simulink model "PV_MEV"  (R2025a)
settings: Solver=VariableStepAuto  StartTime=0.0  StopTime=1  RelTol=1e-3
InitFcn:
  | init_paras
model workspace (MAT data in the model file):
  atk_params = [0 1 0.85 999 0 50 0 0]
  atk_params_vdc = [0 1 0.85 999 0 50 0 0]
values from neighbouring files (symbols this model uses):
  C_PFC = 2600e-6    (= 0.0026)    [init_paras.m]
  ENABLE_HIL = 0    [init_paras.m]
  estimation_src = 1    [init_paras.m]
  Fnom = 50    [init_paras.m]
  Fr_I = Fnom*2    (= 100)    [init_paras.m]
  Ki_V = 80    [init_paras.m]
  Kp_I = 0.06    [init_paras.m]
  Kp_V = 0.25    [init_paras.m]
  Kr_I = 2.5    [init_paras.m]
  L_PFC = 600e-6    (= 0.0006)    [init_paras.m]
  Limit_V = 100    [init_paras.m]
  mm_10cycle_points = mm_points_per_cycle * 10    (= 800)    [init_paras.m]
  mm_fund_freq = 50    [init_paras.m]
  mm_points_per_cycle = 80    [init_paras.m]
  RL_PFC = 20e-3    (= 0.02)    [init_paras.m]
  Ro = 22.22    [init_paras.m]
  Ts_Control = 1/Fc    (= 5e-05)    [init_paras.m]
  Ts_Power = 50e-9    (= 5e-08)    [init_paras.m]
  use_d_predict = 1    [init_paras.m]
  use_harmonic = 1    [init_paras.m]
  use_p_predict = 0    [init_paras.m]
  Vnom_ac = 240    [init_paras.m]
undefined symbols (not defined in the file or in its folder): D1, Delta, DiscIntNeverNeededParam
libraries: spsSeriesRLCBranchLib x17, spsMeanLib x16, spsCurrentMeasurementLib x9, spsFourierLib x8, spsTHDLib x8, spsVoltageMeasurementLib x8, spsDiodeLib x7, MyLibrary x6, instrumentlib x6, pycoexlib x6, simulink x6, spsPWMGeneratorDCDCLib x4
(part 5 of 6)

== system PV_MEV/EV System1/PFC Control/Speed Regulator2 ==
  note: Anti-windup mechanism: Method of conditionnal integration
      |
      | The integration is suspended if saturation occurs and the
      | control error is of the same sign as the control signal.
      |
      | [1] L.Rundqwist, "Anti-Reset Windup for PID Controllers," Ph.D. Thesis TRFT-1033,
      | Departement of Automatic Control, Lund Institute of Technology, Lund, Sweeden, 1991.
  Vref : Inport  PortDimensions=1
  Vmeas : Inport  Port=2  PortDimensions=1
  Add : Sum  Inputs=+|-
  Compare To Zero : simulink/Logic and Bit Operations/Compare To Zero  relop=>  OutDataTypeStr=uint8  ZeroCross=off
  Compare To Zero1 : simulink/Logic and Bit Operations/Compare To Zero  relop=<  OutDataTypeStr=uint8  ZeroCross=off
  Constant : Constant  Value=0
  Constant1 : Constant  Value=Limit_wreg
  Constant2 : Constant  Value=-Limit_wreg
  Discrete-Time Integrator : DiscreteIntegrator  IntegratorMethod=Integration: Trapezoidal  InitialCondition=Init  SampleTime=Ts  LimitOutput=on  UpperSaturationLimit=Limit_wreg  LowerSaturationLimit=-Limit_wreg  ShowStatePort=on  ICPrevOutput=DiscIntNeverNeededParam  ICPrevScaledInput=DiscIntNeverNeededParam
  Kp4 : Gain  Gain=Kp  SaturateOnIntegerOverflow=on  SampleTime=Ts  OutDataTypeStr=Inherit: Same as input  ParamDataTypeStr=Inherit: Same as input
  Kp5 : Gain  Gain=Ki  SaturateOnIntegerOverflow=on  SampleTime=Ts  OutDataTypeStr=Inherit: Same as input  ParamDataTypeStr=Inherit: Same as input
  Logical Operator : Logic  AllPortsSameDT=off  OutDataTypeStr=boolean
  Logical Operator1 : Logic  AllPortsSameDT=off  OutDataTypeStr=boolean
  Logical Operator2 : Logic  Operator=OR  AllPortsSameDT=off  OutDataTypeStr=boolean
  Relational Operator : RelationalOperator  OutDataTypeStr=boolean  InputSameDT=off
  Relational Operator1 : RelationalOperator  Operator=<=  OutDataTypeStr=boolean  InputSameDT=off
  Saturation2 : Saturate  UpperLimit=Limit_wreg  LowerLimit=-Limit_wreg  SampleTime=Ts
  Sum1 : Sum  InputSameDT=on  SaturateOnIntegerOverflow=on  SampleTime=Ts  OutDataTypeStr=Inherit: Same as first input
  Sum6 : Sum  InputSameDT=on  SaturateOnIntegerOverflow=on  SampleTime=Ts  OutDataTypeStr=Inherit: Same as first input
  Switch : Switch  Criteria=u2 > Threshold  SaturateOnIntegerOverflow=off  InputSameDT=off
  Zero-Order Hold : ZeroOrderHold  SampleTime=Ts
  Out : Outport  SampleTime=Ts  InitialOutput=0  VectorParamsAs1DForOutWhenUnconnected=off
  wires:
  Vmeas/1 -> Add/2
  Vref/1 -> Add/1
  Constant/1 -> Switch/1
  Zero-Order Hold/1 -> Sum1/2, Sum6/1
  Discrete-Time Integrator/State -> Sum1/1
  Sum1/1 -> Relational Operator1/1, Relational Operator/1
  Logical Operator2/1 -> Switch/2
  Relational Operator/1 -> Logical Operator/1  "UpperLimit_is_Reached"
  Relational Operator1/1 -> Logical Operator1/1  "LowerLimit_Is_Reached"
  Constant1/1 -> Relational Operator/2
  Constant2/1 -> Relational Operator1/2
  Compare To Zero/1 -> Logical Operator/2  "Error_is_positive"
  Logical Operator/1 -> Logical Operator2/1
  Logical Operator1/1 -> Logical Operator2/2
  Compare To Zero1/1 -> Logical Operator1/2  "Error_is_negative"
  Add/1 -> Kp4/1, Kp5/1, Compare To Zero1/1, Compare To Zero/1
  Sum6/1 -> Saturation2/1
  Kp4/1 -> Zero-Order Hold/1
  Discrete-Time Integrator/1 -> Sum6/2
  Saturation2/1 -> Out/1
  Switch/1 -> Discrete-Time Integrator/1
  Kp5/1 -> Switch/3

== system PV_MEV/EV System1/PFC Control/fft estimation 1 cycle2 ==
  u : Inport
  Buffer 1cycle : Buffer  N=mm_points_per_cycle  V=mm_sampling_overlap  OutputFrames=off
  Constant4 : Constant  Value=mm_fund_freq
  Constant5 : Constant  Value=mm_points_per_cycle * mm_fund_freq
  FFT_estimation_1 : MATLAB Function  TreatAsAtomicUnit=on
  Sampling : ZeroOrderHold  SampleTime=1/(mm_fund_freq*mm_points_per_cycle)
  amp : Outport
  phase : Outport  Port=2
  wires:
  FFT_estimation_1/2(phase) -> phase/1
  FFT_estimation_1/1(amp) -> amp/1
  u/1 -> Sampling/1
  Constant4/1 -> FFT_estimation_1/3(f0)
  Constant5/1 -> FFT_estimation_1/2(fs)
  Buffer 1cycle/1 -> FFT_estimation_1/1(u)
  Sampling/1 -> Buffer 1cycle/1

== system PV_MEV/EV System1/PFC Control/fft estimation 10 cycle2 ==
  u : Inport
  Buffer 10cycle : Buffer  N=mm_10cycle_points  V=mm_10cycle_overlap  OutputFrames=off
  Constant4 : Constant  Value=mm_fund_freq
  Constant5 : Constant  Value=mm_points_per_cycle * mm_fund_freq
  FFT_estimation : MATLAB Function  TreatAsAtomicUnit=on
  Sampling : ZeroOrderHold  SampleTime=1/(mm_fund_freq*mm_points_per_cycle)
  amp : Outport
  phase : Outport  Port=2
  wires:
  Sampling/1 -> Buffer 10cycle/1
  Buffer 10cycle/1 -> FFT_estimation/1(u)
  Constant5/1 -> FFT_estimation/2(fs)
  Constant4/1 -> FFT_estimation/3(f0)
  u/1 -> Sampling/1
  FFT_estimation/1(amp) -> amp/1
  FFT_estimation/2(phase) -> phase/1

== system PV_MEV/EV System2/PFC Control/Half Cycle Model Prediction ==
  u : Inport
  Constant1 : Constant  Value=0.01
  Data Type Conversion : DataTypeConversion  SaturateOnIntegerOverflow=off  RndMeth=Floor
  Data Type Conversion1 : DataTypeConversion  SaturateOnIntegerOverflow=off  RndMeth=Floor
  Data Type Conversion2 : DataTypeConversion  SaturateOnIntegerOverflow=off  RndMeth=Floor
  Demux : Demux  Outputs=7
  MATLAB Function : MATLAB Function  TreatAsAtomicUnit=on
  MATLAB Function3 : MATLAB Function  TreatAsAtomicUnit=on
  Mux1 : Mux  Inputs=3
  Mux6 : Mux
  ONNX Model Predict : pycoexlib/ONNX Model Predict  ModelFile=/home/changhong/prj/finn_cli_fork/scripts/HIL/HarmonicAI_Simulation/Model_Training2/harmonic_brevitas_run_half_opt/brevitas_harmonic_mlp.onnx  ExecutionProviders=CPUExecutionProvider  InputTable={ 'input', 'float32', '', '2' }  OutputTable={ 'output', '', '' }  SampleTime=1/2000  InputDatatypes=float32  InputNumDims=2  InputPermutations=[]  OutputPermutations=[]  PythonCoexecutionBlockType=ONNXModelBlock  VariableOutputMaxSizes=[]
  Sampling1 : ZeroOrderHold  SampleTime=1/2000
  Transpose : Math  Operator=transpose
  u_buff : Buffer  N=40  V=39  OutputFrames=off
  amplitude : Outport
  phase : Outport  Port=2
  wires:
  Transpose/1 -> MATLAB Function/1(x)
  u_buff/1 -> Transpose/1
  u/1 -> Sampling1/1
  Mux1/1 -> phase/1
  Mux6/1 -> amplitude/1
  Data Type Conversion2/1 -> Demux/1
  MATLAB Function3/1(y_post) -> Data Type Conversion2/1
  Demux/1 -> Mux6/1
  Demux/2 -> Mux6/2
  Demux/3 -> Mux6/3
  Demux/4 -> Mux6/4
  Demux/5 -> Mux1/1
  Demux/6 -> Mux1/2
  Demux/7 -> Mux1/3
  MATLAB Function/2(A) -> MATLAB Function3/2(A_latest)
  Constant1/1 -> MATLAB Function3/3(alpha)
  Data Type Conversion1/1 -> MATLAB Function3/1(y_rel)
  ONNX Model Predict/1 -> Data Type Conversion1/1
  Data Type Conversion/1 -> ONNX Model Predict/1
  MATLAB Function/1(x_norm) -> Data Type Conversion/1
  Sampling1/1 -> u_buff/1

== system PV_MEV/EV System2/PFC Control/One  Cycle Model Prediction ==
  u : Inport
  Constant1 : Constant  Value=0.05
  Data Type Conversion : DataTypeConversion  SaturateOnIntegerOverflow=off  RndMeth=Floor
  Data Type Conversion1 : DataTypeConversion  SaturateOnIntegerOverflow=off  RndMeth=Floor
  Data Type Conversion2 : DataTypeConversion  SaturateOnIntegerOverflow=off  RndMeth=Floor
  Demux : Demux  Outputs=7
  MATLAB Function : MATLAB Function  TreatAsAtomicUnit=on
  MATLAB Function3 : MATLAB Function  TreatAsAtomicUnit=on
  Mux1 : Mux  Inputs=3
  Mux6 : Mux
  ONNX Model Predict : pycoexlib/ONNX Model Predict  ModelFile=/home/changhong/prj/finn_cli_fork/scripts/HIL/HarmonicAI_Simulation/Model_Training2/harmonic_brevitas_run_1cycle/brevitas_harmonic_mlp.onnx  ExecutionProviders=AzureExecutionProvider, CPUExecutionProvider  InputTable={ 'input', 'float32', '', '2' }  OutputTable={ 'output', '', '' }  SampleTime=1/4000  InputDatatypes=float32  InputNumDims=2  InputPermutations=[]  OutputPermutations=[]  PythonCoexecutionBlockType=ONNXModelBlock  VariableOutputMaxSizes=[]
  Sampling1 : ZeroOrderHold  SampleTime=1/(mm_fund_freq*mm_points_per_cycle)
  Transpose : Math  Operator=transpose
  u_buff : Buffer  N=mm_points_per_cycle  V=mm_sampling_overlap  OutputFrames=off
  amplitude : Outport
  phase : Outport  Port=2
  wires:
  Sampling1/1 -> u_buff/1
  MATLAB Function/1(x_norm) -> Data Type Conversion/1
  Data Type Conversion/1 -> ONNX Model Predict/1
  ONNX Model Predict/1 -> Data Type Conversion1/1
  Data Type Conversion1/1 -> MATLAB Function3/1(y_rel)
  Constant1/1 -> MATLAB Function3/3(alpha)
  MATLAB Function/2(A) -> MATLAB Function3/2(A_latest)
  Demux/7 -> Mux1/3
  Demux/6 -> Mux1/2
  Demux/5 -> Mux1/1
  Demux/4 -> Mux6/4
  Demux/3 -> Mux6/3
  Demux/2 -> Mux6/2
  Demux/1 -> Mux6/1
  MATLAB Function3/1(y_post) -> Data Type Conversion2/1
  Data Type Conversion2/1 -> Demux/1
  Mux6/1 -> amplitude/1
  Mux1/1 -> phase/1
  u/1 -> Sampling1/1
  u_buff/1 -> Transpose/1
  Transpose/1 -> MATLAB Function/1(x)

== system PV_MEV/EV System2/PFC Control/PR2 ==
  Iref : Inport
  Iac : Inport  Port=2
  Gain : Gain  Gain=Kp
  Gain1 : Gain  Gain=Kr
  Second-Order Filter1 : spsSecondOrderFilterLib/Second-Order Filter  FilterType=Bandpass  Fo=Fr  Zeta=Zeta_I  Ts=Ts_Control  Initialize=off  Vac_Init="[0,  0,  60]"  Vdc_Init=0  PlotResponse=off  FreqRange=[0, 1000, 0.2]
  Sum1 : Sum  Inputs=|+-
  Sum2 : Sum  Inputs=|++
  D : Outport
  wires:
  Gain1/1 -> Second-Order Filter1/1
  Sum2/1 -> D/1
  Gain/1 -> Sum2/1
  Iac/1 -> Sum1/2
  Iref/1 -> Sum1/1
  Sum1/1 -> Gain1/1, Gain/1
  Second-Order Filter1/1 -> Sum2/2

== system PV_MEV/EV System2/PFC Control/Speed Regulator2 ==
  note: Anti-windup mechanism: Method of conditionnal integration
      |
      | The integration is suspended if saturation occurs and the
      | control error is of the same sign as the control signal.
      |
      | [1] L.Rundqwist, "Anti-Reset Windup for PID Controllers," Ph.D. Thesis TRFT-1033,
      | Departement of Automatic Control, Lund Institute of Technology, Lund, Sweeden, 1991.
  Vref : Inport  PortDimensions=1
  Vmeas : Inport  Port=2  PortDimensions=1
  Add : Sum  Inputs=+|-
  Compare To Zero : simulink/Logic and Bit Operations/Compare To Zero  relop=>  OutDataTypeStr=uint8  ZeroCross=off
  Compare To Zero1 : simulink/Logic and Bit Operations/Compare To Zero  relop=<  OutDataTypeStr=uint8  ZeroCross=off
  Constant : Constant  Value=0
  Constant1 : Constant  Value=Limit_wreg
  Constant2 : Constant  Value=-Limit_wreg
  Discrete-Time Integrator : DiscreteIntegrator  IntegratorMethod=Integration: Trapezoidal  InitialCondition=Init  SampleTime=Ts  LimitOutput=on  UpperSaturationLimit=Limit_wreg  LowerSaturationLimit=-Limit_wreg  ShowStatePort=on  ICPrevOutput=DiscIntNeverNeededParam  ICPrevScaledInput=DiscIntNeverNeededParam
  Kp4 : Gain  Gain=Kp  SaturateOnIntegerOverflow=on  SampleTime=Ts  OutDataTypeStr=Inherit: Same as input  ParamDataTypeStr=Inherit: Same as input
  Kp5 : Gain  Gain=Ki  SaturateOnIntegerOverflow=on  SampleTime=Ts  OutDataTypeStr=Inherit: Same as input  ParamDataTypeStr=Inherit: Same as input
  Logical Operator : Logic  AllPortsSameDT=off  OutDataTypeStr=boolean
  Logical Operator1 : Logic  AllPortsSameDT=off  OutDataTypeStr=boolean
  Logical Operator2 : Logic  Operator=OR  AllPortsSameDT=off  OutDataTypeStr=boolean
  Relational Operator : RelationalOperator  OutDataTypeStr=boolean  InputSameDT=off
  Relational Operator1 : RelationalOperator  Operator=<=  OutDataTypeStr=boolean  InputSameDT=off
  Saturation2 : Saturate  UpperLimit=Limit_wreg  LowerLimit=-Limit_wreg  SampleTime=Ts
  Sum1 : Sum  InputSameDT=on  SaturateOnIntegerOverflow=on  SampleTime=Ts  OutDataTypeStr=Inherit: Same as first input
  Sum6 : Sum  InputSameDT=on  SaturateOnIntegerOverflow=on  SampleTime=Ts  OutDataTypeStr=Inherit: Same as first input
  Switch : Switch  Criteria=u2 > Threshold  SaturateOnIntegerOverflow=off  InputSameDT=off
  Zero-Order Hold : ZeroOrderHold  SampleTime=Ts
  Out : Outport  SampleTime=Ts  InitialOutput=0  VectorParamsAs1DForOutWhenUnconnected=off
  wires:
  Kp5/1 -> Switch/3
  Switch/1 -> Discrete-Time Integrator/1
  Saturation2/1 -> Out/1
  Discrete-Time Integrator/1 -> Sum6/2
  Kp4/1 -> Zero-Order Hold/1
  Sum6/1 -> Saturation2/1
  Add/1 -> Compare To Zero/1, Compare To Zero1/1, Kp5/1, Kp4/1
  Compare To Zero1/1 -> Logical Operator1/2  "Error_is_negative"
  Logical Operator1/1 -> Logical Operator2/2
  Logical Operator/1 -> Logical Operator2/1
  Compare To Zero/1 -> Logical Operator/2  "Error_is_positive"
  Constant2/1 -> Relational Operator1/2
  Constant1/1 -> Relational Operator/2
  Relational Operator1/1 -> Logical Operator1/1  "LowerLimit_Is_Reached"
  Relational Operator/1 -> Logical Operator/1  "UpperLimit_is_Reached"
  Logical Operator2/1 -> Switch/2
  Sum1/1 -> Relational Operator/1, Relational Operator1/1
  Discrete-Time Integrator/State -> Sum1/1
  Zero-Order Hold/1 -> Sum6/1, Sum1/2
  Constant/1 -> Switch/1
  Vref/1 -> Add/1
  Vmeas/1 -> Add/2

== system PV_MEV/EV System2/PFC Control/fft estimation 1 cycle2 ==
  u : Inport
  Buffer 1cycle : Buffer  N=mm_points_per_cycle  V=mm_sampling_overlap  OutputFrames=off
  Constant4 : Constant  Value=mm_fund_freq
  Constant5 : Constant  Value=mm_points_per_cycle * mm_fund_freq
  FFT_estimation_1 : MATLAB Function  TreatAsAtomicUnit=on
  Sampling : ZeroOrderHold  SampleTime=1/(mm_fund_freq*mm_points_per_cycle)
  amp : Outport
  phase : Outport  Port=2
  wires:
  Sampling/1 -> Buffer 1cycle/1
  Buffer 1cycle/1 -> FFT_estimation_1/1(u)
  Constant5/1 -> FFT_estimation_1/2(fs)
  Constant4/1 -> FFT_estimation_1/3(f0)
  u/1 -> Sampling/1
  FFT_estimation_1/1(amp) -> amp/1
  FFT_estimation_1/2(phase) -> phase/1

== system PV_MEV/EV System2/PFC Control/fft estimation 10 cycle2 ==
  u : Inport
  Buffer 10cycle : Buffer  N=mm_10cycle_points  V=mm_10cycle_overlap  OutputFrames=off
  Constant4 : Constant  Value=mm_fund_freq
  Constant5 : Constant  Value=mm_points_per_cycle * mm_fund_freq
  FFT_estimation : MATLAB Function  TreatAsAtomicUnit=on
  Sampling : ZeroOrderHold  SampleTime=1/(mm_fund_freq*mm_points_per_cycle)
  amp : Outport
  phase : Outport  Port=2
  wires:
  FFT_estimation/2(phase) -> phase/1
  FFT_estimation/1(amp) -> amp/1
  u/1 -> Sampling/1
  Constant4/1 -> FFT_estimation/3(f0)
  Constant5/1 -> FFT_estimation/2(fs)
  Buffer 10cycle/1 -> FFT_estimation/1(u)
  Sampling/1 -> Buffer 10cycle/1

== system PV_MEV/PV System/DC AC Inverter/VSC Control ==
  note: VSC Main Controller
  Vabc_prim : Inport  PortDimensions=3
  Iabc_prim : Inport  Port=2  PortDimensions=3
  Vdc_mes : Inport  Port=3  PortDimensions=1
  Current Regulator : Subsystem
  Iq_ref : Constant  Value=0
  Mux : Mux  Inputs=2
  PLL & Measurements : Subsystem
  PWM Generator (3-Level) : spsPWMGenerator3LevelLib/PWM Generator (3-Level)  ModulatorType=Three-phase bridge (12 pulses)  ModulatorMode=Unsynchronized  nF=27  Fc=33*60  ModulatingSignals=off  m=0.8  Freq=60  Phase=0  Ts=Ts_Power
  Uabc_ref Generation max (m) = 1 : Subsystem
  Unit Delay : UnitDelay  SampleTime=Ts_Control  HasFrameUpgradeWarning=on
  VDC Regulator : Subsystem
  Vdc_ref1 : Constant  Value=Vdc_ref
  Pulses : Outport  VectorParamsAs1DForOutWhenUnconnected=off
  wires:
  VDC Regulator/1(Id_ref) -> Mux/1
  PLL & Measurements/1(wt) -> Uabc_ref Generation max (m) = 1/1(wt)
  Current Regulator/1(VdVq_conv) -> Uabc_ref Generation max (m) = 1/2(VdVq_conv)
  Iq_ref/1 -> Mux/2
  Mux/1 -> Current Regulator/3(IdIq_ref)
  PLL & Measurements/3(IdIq_prim) -> Current Regulator/2(IdIq_mes)
  PLL & Measurements/2(VdVq_prim) -> Current Regulator/1(VdVq_mes)
  Vdc_mes/1 -> VDC Regulator/1(Vdc_mes)
  Vabc_prim/1 -> PLL & Measurements/1(Vabc_prim)
  Iabc_prim/1 -> PLL & Measurements/2(Iabc_prim)
  Unit Delay/1 -> PWM Generator (3-Level)/1
  PWM Generator (3-Level)/1 -> Pulses/1
  Uabc_ref Generation max (m) = 1/1(Uabc_ref) -> Unit Delay/1
  Vdc_ref1/1 -> VDC Regulator/2(Vdc_ref)

== system PV_MEV/PV System/DC DC Boost Converter/MPPT Controller using  'Incremental Conductance + Integral Regulator'  technique  ==
  V_PV : Inport
  I_PV : Inport  Port=2
  Add : Sum  Inputs=+-
  Deblock MPPT : Step  Time=0.4  SampleTime=0
  Duty Cycle : Constant  Value=Dinit
  MPPT : Subsystem
  PWM Generator (DC-DC) : spsPWMGeneratorDCDCLib/PWM Generator (DC-DC)  Fsw=fc  Ts=Ts_Power
  Saturation : Saturate  UpperLimit=1  LowerLimit=0
  Pulses : Outport  VectorParamsAs1DForOutWhenUnconnected=off
  tag scope: D=global
  wires:
  V_PV/1 -> MPPT/1(V_PV)
  I_PV/1 -> MPPT/2(I_PV)
  PWM Generator (DC-DC)/1 -> Pulses/1
  Deblock MPPT/1 -> MPPT/3(on/off)
  Saturation/1 -> PWM Generator (DC-DC)/1, [D]
  Add/1 -> Saturation/1  "D"
  MPPT/1(Delta_D) -> Add/2
  Duty Cycle/1 -> Add/1

== system PV_MEV/PV System/DC AC Inverter/VSC Control/Current Regulator ==
  note: harmonic filter neglected
  note: Vd_mes + Id*R - Iq*L + deriv(Id)*L= Vd_conv
  note: Vq_mes + Id*L + Iq*R + deriv(Iq)*L= Vq_conv
  note: Current Regulator
      | (with feedforward)
  note: Sign Convention: Current going out of the converter = positive current
  note: Iq positive --> The converter absorbs reactive power ("Inductive mode") = Reactive Power Q negative
  note: Id positive --> The converter generates active power ("Inverter mode") = Active Power P positive
  note: Ltot = Lxfo + Lchoke
      | Rtot = Rxfo + Rchoke
  note: (Vd_prim - Vd_conv) ~= + Iq * Ltot
  note: (Vq_prim - Vq_conv) ~ = - Id * Ltot
  note: For Ltot >> Rtot :
  VdVq_mes : Inport  PortDimensions=2
  IdIq_mes : Inport  Port=2  PortDimensions=2
  IdIq_ref : Inport  Port=3  PortDimensions=2
  Add1 : Sum  Inputs=++-
  Add2 : Sum
  Add3 : Sum  Inputs=+++
  Demux : Demux  Outputs=2
  Demux1 : Demux  Outputs=2
  Ltot_pu1 : Gain  Gain=Ltot_pu  SaturateOnIntegerOverflow=on  OutDataTypeStr=Inherit: Same as input  ParamDataTypeStr=Inherit: Same as input
  Ltot_pu2 : Gain  Gain=Ltot_pu  SaturateOnIntegerOverflow=on  OutDataTypeStr=Inherit: Same as input  ParamDataTypeStr=Inherit: Same as input
  Mux : Mux  Inputs=2
  PI : slpidlib/PID Controller  Controller=PI  Form=Parallel  TimeDomain=Discrete-time  UseExternalTs=off  SampleTime=Ts  IntegratorMethod=Forward Euler  FilterMethod=Forward Euler  ControllerParametersSource=internal  P=Kp_Ireg  I=Ki_Ireg  UseKiTs=off  D=0  UseExternalDerivativeSource=off  N=100  UseFilter=on  TunerSelectOption=Transfer Function Based (PID Tuner App)  InitialConditionSource=internal  InitialConditionForIntegrator=0  InitialConditionForFilter=0  DifferentiatorICPrevScaledInput=0  ExternalReset=none  TrackingMode=off  Kt=1  LimitOutput=on  SatLimitsSource=internal  UpperSaturationLimit=2  LowerSaturationLimit=-2  LinearizeAsGain=off  AntiWindupMode=none  Kb=1  LimitIntegrator=off  UpperIntegratorSaturationLimit=inf  LowerIntegratorSaturationLimit=-inf  POutMin=[]  POutMax=[]  IOutMin=[]  IOutMax=[]  DOutMin=[]  DOutMax=[]  NOutMin=[]  NOutMax=[]  SumOutMin=[]  SumOutMax=[]  SaturationOutMin=[]  SaturationOutMax=[]  PParamMin=[]  PParamMax=[]  IParamMin=[]  IParamMax=[]  DParamMin=[]  DParamMax=[]  NParamMin=[]  NParamMax=[]  KbParamMin=[]  KbParamMax=[]  KtParamMin=[]  KtParamMax=[]  KbOutMin=[]  KbOutMax=[]  KtOutMin=[]  KtOutMax=[]  IntegratorOutMin=[]  IntegratorOutMax=[]  FilterOutMin=[]  FilterOutMax=[]  SumI1OutMin=[]  SumI1OutMax=[]  SumI2OutMin=[]  SumI2OutMax=[]  SumI3OutMin=[]  SumI3OutMax=[]  SumI4OutMin=[]  SumI4OutMax=[]  SumDOutMin=[]  SumDOutMax=[]  DifferentiatorOutMin=[]  DifferentiatorOutMax=[]  FilterDiffOutCoefMin=[]  FilterDiffOutCoefMax=[]  ReciprocalOutMin=[]  ReciprocalOutMax=[]  SumDenOutMin=[]  SumDenOutMax=[]  SumNumOutMin=[]  SumNumOutMax=[]  DivideOutMin=[]  DivideOutMax=[]  UdiffTsProdOutMin=[]  UdiffTsProdOutMax=[]  NTsProdOutMin=[]  NTsProdOutMax=[]  UintegralTsProdOutMin=[]  UintegralTsProdOutMax=[]  UngainTsProdOutMin=[]  UngainTsProdOutMax=[]  ClampingZeroOutDataTypeStr=Inherit: Inherit via back propagation  ClampingZeroOutMin=[]  ClampingZeroOutMax=[]  FilterDenConstantOutDataTypeStr=Inherit: Inherit via back propagation  FilterDenConstantOutMin=[]  FilterDenConstantOutMax=[]  PCopyOutDataTypeStr=Inherit: Inherit via back propagation  PCopyOutMin=[]  PCopyOutMax=[]  NCopyOutDataTypeStr=Inherit: Inherit via back propagation  NCopyOutMin=[]  NCopyOutMax=[]  IntegratorContinuousStateAttributes=''  IntegratorStateMustResolveToSignalObject=off  IntegratorRTWStateStorageClass=Auto  FilterContinuousStateAttributes=''  FilterStateMustResolveToSignalObject=off  FilterRTWStateStorageClass=Auto  ParallelPVariant=InternalParameters  IdealPVariant=Disabled  IVariant=InternalParameters  DVariant=Disabled  IntegratorVariant=Discrete  SatVariant=Enabled  AWVariant=Passthrough  PCopyVariant=Disabled  TRVariant=Disabled  FdbkBlocksVariant=Forward  IdealPFdbkVariant=Disabled  SatFdbkVariant=Disabled  DerivativeFilterVariant=Disabled  NVariant=Disabled  NCopyVariant=Disabled_SignalSpec  FilterICVariant=Disabled  IntegratorICVariant=InternalICs  ExternalResetVariant=Disabled  TRSumVariant=Passthrough  SumFdbkVariant=Disabled  SumVariant=Sum_PI  TsampFilterVariant=InternalTs  TsampNgainVariant=Passthrough  TsampIntegralVariant=Disabled_SignalSpec  ExternalSaturationOutDataTypeStr=Inherit: Same as second input  DerivativeSourceVariant=Disabled  PreIntVariant=InternalPreInt
  PI_Ireg1 : Scope
      settings: DataLoggingSaveFormat=Array
  Rtot_pu1 : Gain  Gain=Rtot_pu  SaturateOnIntegerOverflow=on  OutDataTypeStr=Inherit: Same as input  ParamDataTypeStr=Inherit: Same as input
  Rtot_pu5 : Gain  Gain=Rtot_pu  SaturateOnIntegerOverflow=on  OutDataTypeStr=Inherit: Same as input  ParamDataTypeStr=Inherit: Same as input
  Saturation : Saturate  UpperLimit=2  LowerLimit=-2
  Sum : Sum  Inputs=|-+
  VdVq_conv : Outport  VectorParamsAs1DForOutWhenUnconnected=off
  wires:
  Mux/1 -> PI_Ireg1/1, Add2/2
  PI/1 -> Add2/1  "PI"
  Sum/1 -> PI/1
  IdIq_ref/1 -> Sum/2, Demux1/1
  IdIq_mes/1 -> Sum/1
  Add2/1 -> Saturation/1
  Saturation/1 -> VdVq_conv/1
  VdVq_mes/1 -> Demux/1
  Demux/1 -> Add1/1
  Rtot_pu1/1 -> Add1/2
  Demux1/1 -> Rtot_pu1/1, Ltot_pu2/1
  Ltot_pu1/1 -> Add1/3
  Demux1/2 -> Ltot_pu1/1, Rtot_pu5/1
  Rtot_pu5/1 -> Add3/2
  Ltot_pu2/1 -> Add3/3
  Add1/1 -> Mux/1  "Feedforward"
  Demux/2 -> Add3/1
  Add3/1 -> Mux/2

== system PV_MEV/PV System/DC AC Inverter/VSC Control/PLL & Measurements ==
  Vabc_prim : Inport
  Iabc_prim : Inport  Port=2
  PLL (3ph) : spsPLL3phLib/PLL (3ph)  Fmin=45  Par_Init="[-0.57  Fnom]"  ParK=[180, 3200, 1]  TcD=1e-4  MaxRateChangeFreq=12  FilterCutOffFreq=25  Ts=Ts  AGC=on
  Selector1 : Selector  InputPortWidth=3  IndexOptions=Index vector (dialog)  Indices=[1 2]  OutputSizes=1
  Selector2 : Selector  InputPortWidth=3  IndexOptions=Index vector (dialog)  Indices=[1 2]  OutputSizes=1
  Terminator : Terminator
  V->pu : Gain  Gain=1/(Vnom_prim*sqrt(2)/sqrt(3))  SaturateOnIntegerOverflow=on  OutDataTypeStr=Inherit: Same as input  ParamDataTypeStr=Inherit: Same as input
  V->pu1 : Gain  Gain=Vnom_prim*sqrt(3)/Pnom/sqrt(2)  SaturateOnIntegerOverflow=on  OutDataTypeStr=Inherit: Same as input  ParamDataTypeStr=Inherit: Same as input
  abc to dq0 : spsabctodq0Lib/abc to dq0  Alignment=90 degrees behind phase A axis
  abc to dq1 : spsabctodq0Lib/abc to dq0  Alignment=90 degrees behind phase A axis
  wt : Outport  VectorParamsAs1DForOutWhenUnconnected=off
  VdVq_prim : Outport  Port=2  VectorParamsAs1DForOutWhenUnconnected=off
  IdIq_prim : Outport  Port=3  VectorParamsAs1DForOutWhenUnconnected=off
  tag scope: IdIq_prim=global
  wires:
  V->pu1/1 -> abc to dq1/1
  V->pu/1 -> PLL (3ph)/1, abc to dq0/1
  abc to dq1/1 -> Selector1/1
  Vabc_prim/1 -> V->pu/1
  Iabc_prim/1 -> V->pu1/1
  abc to dq0/1 -> Selector2/1
  Selector2/1 -> VdVq_prim/1
  Selector1/1 -> [IdIq_prim], IdIq_prim/1
  PLL (3ph)/2 -> wt/1, abc to dq1/2, abc to dq0/2
  PLL (3ph)/1 -> Terminator/1

== system PV_MEV/PV System/DC AC Inverter/VSC Control/Uabc_ref Generation max (m) = 1 ==
  note: (Correction for transformer
      |  D1 connection)
  note: (Correction for delai of Ts_Control)
  wt : Inport
  VdVq_conv : Inport  Port=2
  Add1 : Sum  Inputs=++++
  Add2 : Sum
  Complex to Magnitude-Angle : ComplexToMagnitudeAngle
  Constant : Constant  Value=-pi/6
  Constant1 : Constant  Value=Vnom_dc
  Constant2 : Constant  Value="[ 0  -2*pi/3  2*pi/3  ]"
  Constant3 : Constant  Value=Vnom_sec*sqrt(2)/sqrt(3)
  Constant4 : Constant  Value=Ts*Fnom*(2*pi)
  Demux1 : Demux  Outputs=2
  Gain1 : Gain  Gain=1/2
  Product : Product  Inputs=*/  RndMeth=Zero
  Product1 : Product  Inputs=*/  RndMeth=Zero
  Product2 : Product  Inputs=**  RndMeth=Zero
  Real-Imag to Complex : RealImagToComplex
  Saturation : Saturate  UpperLimit=1  LowerLimit=0
  Trigonometric Function : Trigonometry
  Uabc_ref : Outport  VectorParamsAs1DForOutWhenUnconnected=off
  tag scope: m=global
  wires:
  Complex to Magnitude-Angle/1 -> Saturation/1
  Constant1/1 -> Gain1/1
  VdVq_conv/1 -> Product1/1
  Product1/1 -> Demux1/1
  Gain1/1 -> Product/1
  Real-Imag to Complex/1 -> Complex to Magnitude-Angle/1
  Demux1/1 -> Real-Imag to Complex/1
  Demux1/2 -> Real-Imag to Complex/2
  Constant2/1 -> Add1/2
  Constant/1 -> Add1/3
  Constant3/1 -> Product/2
  Product/1 -> Product1/2
  Complex to Magnitude-Angle/2 -> Add2/1
  Add1/1 -> Add2/2
  Add2/1 -> Trigonometric Function/1
  Saturation/1 -> [m], Product2/1
  Trigonometric Function/1 -> Product2/2
  Product2/1 -> Uabc_ref/1
  wt/1 -> Add1/1
  Constant4/1 -> Add1/4

== system PV_MEV/PV System/DC AC Inverter/VSC Control/VDC Regulator ==
  Vdc_mes : Inport  PortDimensions=1
  Vdc_ref : Inport  Port=2  PortDimensions=1
  PI : slpidlib/PID Controller  Controller=PI  Form=Parallel  TimeDomain=Discrete-time  UseExternalTs=off  SampleTime=Ts  IntegratorMethod=Trapezoidal  FilterMethod=Forward Euler  ControllerParametersSource=internal  P=Kp_VDCreg  I=Ki_VDCreg  UseKiTs=off  D=0  UseExternalDerivativeSource=off  N=100  UseFilter=on  TunerSelectOption=Transfer Function Based (PID Tuner App)  InitialConditionSource=internal  InitialConditionForIntegrator=0  InitialConditionForFilter=0  DifferentiatorICPrevScaledInput=0  ExternalReset=none  TrackingMode=off  Kt=1  LimitOutput=on  SatLimitsSource=internal  UpperSaturationLimit=1.5  LowerSaturationLimit=-1.5  LinearizeAsGain=off  AntiWindupMode=none  Kb=1  LimitIntegrator=off  UpperIntegratorSaturationLimit=inf  LowerIntegratorSaturationLimit=-inf  POutMin=[]  POutMax=[]  IOutMin=[]  IOutMax=[]  DOutMin=[]  DOutMax=[]  NOutMin=[]  NOutMax=[]  SumOutMin=[]  SumOutMax=[]  SaturationOutMin=[]  SaturationOutMax=[]  PParamMin=[]  PParamMax=[]  IParamMin=[]  IParamMax=[]  DParamMin=[]  DParamMax=[]  NParamMin=[]  NParamMax=[]  KbParamMin=[]  KbParamMax=[]  KtParamMin=[]  KtParamMax=[]  KbOutMin=[]  KbOutMax=[]  KtOutMin=[]  KtOutMax=[]  IntegratorOutMin=[]  IntegratorOutMax=[]  FilterOutMin=[]  FilterOutMax=[]  SumI1OutMin=[]  SumI1OutMax=[]  SumI2OutMin=[]  SumI2OutMax=[]  SumI3OutMin=[]  SumI3OutMax=[]  SumI4OutMin=[]  SumI4OutMax=[]  SumDOutMin=[]  SumDOutMax=[]  DifferentiatorOutMin=[]  DifferentiatorOutMax=[]  FilterDiffOutCoefMin=[]  FilterDiffOutCoefMax=[]  ReciprocalOutMin=[]  ReciprocalOutMax=[]  SumDenOutMin=[]  SumDenOutMax=[]  SumNumOutMin=[]  SumNumOutMax=[]  DivideOutMin=[]  DivideOutMax=[]  UdiffTsProdOutMin=[]  UdiffTsProdOutMax=[]  NTsProdOutMin=[]  NTsProdOutMax=[]  UintegralTsProdOutMin=[]  UintegralTsProdOutMax=[]  UngainTsProdOutMin=[]  UngainTsProdOutMax=[]  ClampingZeroOutDataTypeStr=Inherit: Inherit via back propagation  ClampingZeroOutMin=[]  ClampingZeroOutMax=[]  FilterDenConstantOutDataTypeStr=Inherit: Inherit via back propagation  FilterDenConstantOutMin=[]  FilterDenConstantOutMax=[]  PCopyOutDataTypeStr=Inherit: Inherit via back propagation  PCopyOutMin=[]  PCopyOutMax=[]  NCopyOutDataTypeStr=Inherit: Inherit via back propagation  NCopyOutMin=[]  NCopyOutMax=[]  IntegratorContinuousStateAttributes=''  IntegratorStateMustResolveToSignalObject=off  IntegratorRTWStateStorageClass=Auto  FilterContinuousStateAttributes=''  FilterStateMustResolveToSignalObject=off  FilterRTWStateStorageClass=Auto  ParallelPVariant=InternalParameters  IdealPVariant=Disabled  IVariant=InternalParameters  DVariant=Disabled  IntegratorVariant=Discrete  SatVariant=Enabled  AWVariant=Passthrough  PCopyVariant=Disabled  TRVariant=Disabled  FdbkBlocksVariant=Forward  IdealPFdbkVariant=Disabled  SatFdbkVariant=Disabled  DerivativeFilterVariant=Disabled  NVariant=Disabled  NCopyVariant=Disabled_SignalSpec  FilterICVariant=Disabled  IntegratorICVariant=InternalICs  ExternalResetVariant=Disabled  TRSumVariant=Passthrough  SumFdbkVariant=Disabled  SumVariant=Sum_PI  TsampFilterVariant=InternalTs  TsampNgainVariant=Passthrough  TsampIntegralVariant=Disabled_SignalSpec  ExternalSaturationOutDataTypeStr=Inherit: Same as second input  DerivativeSourceVariant=Disabled  PreIntVariant=InternalPreInt
  Rtot_pu3 : Gain  Gain=1/Vnom_dc  SaturateOnIntegerOverflow=on  OutDataTypeStr=Inherit: Same as input  ParamDataTypeStr=Inherit: Same as input
  Sum : Sum  Inputs=|+-
  Id_ref : Outport  SampleTime=Ts  InitialOutput=0  VectorParamsAs1DForOutWhenUnconnected=off
  tag scope: Id_ref=global, Vdc_ref=global
  wires:
  Sum/1 -> Rtot_pu3/1
  Vdc_mes/1 -> Sum/1
  Vdc_ref/1 -> Sum/2, [Vdc_ref]
  Rtot_pu3/1 -> PI/1
  PI/1 -> [Id_ref], Id_ref/1

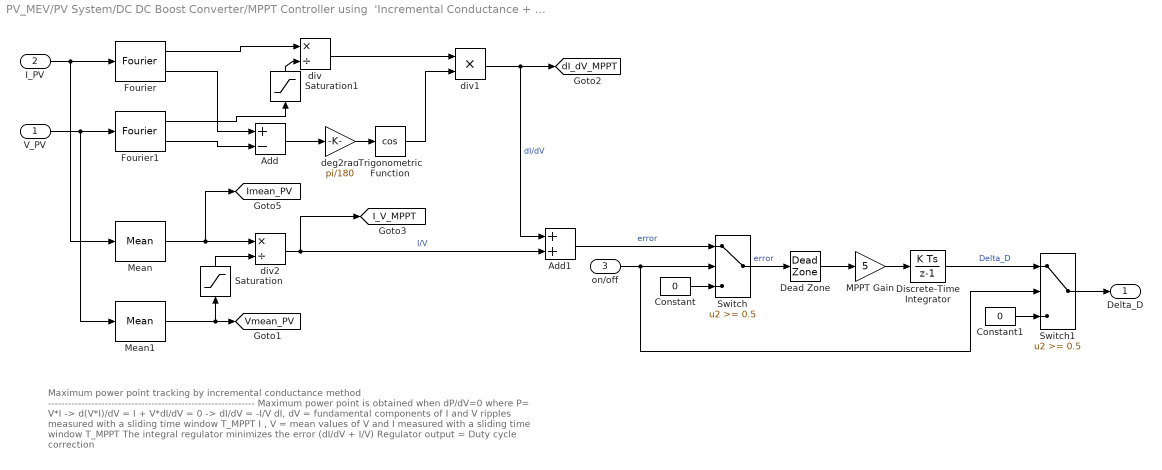
== system PV_MEV/PV System/DC DC Boost Converter/MPPT Controller using  'Incremental Conductance + Integral Regulator'  technique /MPPT ==
  note: Maximum power point tracking by incremental conductance method
      | --------------------------------------------------------------
      | Maximum power point is obtained when dP/dV=0  where P= V*I
      | -> d(V*I)/dV = I + V*dI/dV = 0
      | -> dI/dV = -I/V
      |
      | dI, dV  = fundamental components of I and V ripples measured with a sliding time window T_MPPT
      | I , V   = mean values of V and I measured with a sliding time window T_MPPT
      |
      | The integral regulator minimizes the error (dI/dV + I/V)
      | Regulator output = Duty cycle correction
  V_PV : Inport
  I_PV : Inport  Port=2
  on/off : Inport  Port=3
  Add : Sum  Inputs=+-
  Add1 : Sum
  Constant : Constant  Value=0
  Constant1 : Constant  Value=0
  Dead Zone : DeadZone  LowerValue=-0.05  UpperValue=0.05
  Discrete-Time Integrator : DiscreteIntegrator  SampleTime=Ts_Control  LimitOutput=on  UpperSaturationLimit=1  LowerSaturationLimit=-1  ICPrevOutput=DiscIntNeverNeededParam  ICPrevScaledInput=DiscIntNeverNeededParam
  Fourier : spsFourierLib/Fourier  Freq=1/T_MPPT  n=1  InInit=[0, 0]  Ts=Ts_Control
  Fourier1 : spsFourierLib/Fourier  Freq=1/T_MPPT  n=1  InInit=[0, 0]  Ts=Ts_Control
  MPPT Gain : Gain  Gain=5
  Mean : spsMeanLib/Mean  Freq=1/T_MPPT  Vinit=0  Ts=Ts_Control
  Mean1 : spsMeanLib/Mean  Freq=1/T_MPPT  Vinit=0  Ts=Ts_Control
  Saturation : Saturate  UpperLimit=inf  LowerLimit=eps
  Saturation1 : Saturate  UpperLimit=inf  LowerLimit=eps
  Switch : Switch  Threshold=0.5  SaturateOnIntegerOverflow=off  InputSameDT=off
  Switch1 : Switch  Threshold=0.5  SaturateOnIntegerOverflow=off  InputSameDT=off
  Trigonometric Function : Trigonometry  Operator=cos
  deg2rad : Gain  Gain=pi/180
  div : Product  Inputs=*/  RndMeth=Zero
  div1 : Product  Inputs=**  RndMeth=Zero
  div2 : Product  Inputs=*/  RndMeth=Zero
  Delta_D : Outport  VectorParamsAs1DForOutWhenUnconnected=off
  tag scope: I_V_MPPT=global, Imean_PV=global, Vmean_PV=global, dI_dV_MPPT=global
  wires:
  Dead Zone/1 -> MPPT Gain/1
  Switch/1 -> Dead Zone/1  "error"
  Saturation1/1 -> div/2
  Saturation/1 -> div2/2
  Switch1/1 -> Delta_D/1
  on/off/1 -> Switch/2, Switch1/2
  Constant1/1 -> Switch1/3
  Discrete-Time Integrator/1 -> Switch1/1  "Delta_D"
  Constant/1 -> Switch/3
  MPPT Gain/1 -> Discrete-Time Integrator/1
  Add1/1 -> Switch/1  "error"
  div2/1 -> Add1/2, [I_V_MPPT]  "I/V"
  Mean1/1 -> Saturation/1, [Vmean_PV]
  Mean/1 -> div2/1, [Imean_PV]
  div1/1 -> Add1/1, [dI_dV_MPPT]  "dI/dV"
  Trigonometric Function/1 -> div1/2
  div/1 -> div1/1
  deg2rad/1 -> Trigonometric Function/1
  Add/1 -> deg2rad/1
  Fourier1/1 -> Saturation1/1
  Fourier1/2 -> Add/2
  Fourier/2 -> Add/1
  V_PV/1 -> Mean1/1, Fourier1/1
  I_PV/1 -> Mean/1, Fourier/1
  Fourier/1 -> div/1

== matlab function PV_MEV/EV System1/PFC Control/D_predict ==
  data: i_L input; D output; i_ref input; V_in input; Ts input; L_in input; V_o input; theta_pll input; amp_est input; phase_est input; use_harmonic input
function D  = fcn(i_L, i_ref, V_in, Ts, L_in, V_o, theta_pll, amp_est, phase_est, use_harmonic)

    persistent theta_prev;
    if isempty(theta_prev)
        theta_prev = theta_pll;
    end

    % hyper parameters
    track_gain = 0.35;
    damp_gain = 0.015;

    % Optional
    lead_steps = 1.0;


    % Initialisation 
    L = max(L_in, 1e-9);
    Ts_eff = max(Ts, 1e-9);
    Vo = max(abs(V_o), 1.0);
    ui_L = abs(i_L);

    if V_in > 0
        line_sign = 1.0;
    else
        line_sign = -1.0;
    end

    i_ref_signed = line_sign * abs(i_ref);

    plant_gain = line_sign * L / (Vo * Ts_eff);
    D_ff = 1.0 - abs(V_in) / Vo;

    if use_harmonic

        dtheta = atan2(sin(theta_pll - theta_prev), cos(theta_pll - theta_prev));
        theta_prev = theta_pll;

        omega_inst = dtheta / Ts_eff;

        theta_ctrl = theta_pll + omega_inst * Ts_eff * lead_steps;

        A3 = abs(amp_est(2));
        A5 = abs(amp_est(3));
        A7 = abs(amp_est(4));

        phi3 = phase_est(1);
        phi5 = phase_est(2);
        phi7 = phase_est(3);

        phase_sign = 1.0;

        ih3 = A3 * sin(3.0 * theta_ctrl + phase_sign * phi3);
        ih5 = A5 * sin(5.0 * theta_ctrl + phase_sign * phi5);
        ih7 = A7 * sin(7.0 * theta_ctrl + phase_sign * phi7);

        k3 = 1.00;
        k5 = 1.08;
        k7 = 1.00;

        ih_357 = k3 * ih3 + k5 * ih5 + k7 * ih7;

        i_ref_signed = i_ref_signed - ih_357;
    end

    i_err = i_ref_signed - i_L;

    D_corr = plant_gain * track_gain * i_err;
    D_damp = -line_sign * damp_gain * (i_L - i_ref_signed) / ui_L;

    D = D_ff + D_corr + D_damp;
end

== matlab function PV_MEV/EV System1/PFC Control/Half Cycle Model Prediction/MATLAB Function ==
  data: x input; x_norm output; A output
function [x_norm, A] = CycleNorm(x)
A = max(abs(x));
A = max(A, 1e-6);
x_norm = x / A;

== matlab function PV_MEV/EV System1/PFC Control/Half Cycle Model Prediction/MATLAB Function3 ==
  data: y_rel input; y_post output; A_latest input; alpha input; reset input
function y_post = harmonic_postprocess(y_rel, A_latest, alpha, reset)
%#codegen
% 一体化后处理：
% 1) EMA 平滑（在相对输出域）
% 2) A 恢复（幅值乘 A）
% 3) atan2 恢复相位（由 cos/sin -> phase）
%
% 输入:
%   y_rel    : 模型输出(10x1 或 1x10)
%              [amp_h1_rel, amp_h3_rel, amp_h5_rel, amp_h7_rel, ...
%               cos_h3, sin_h3, cos_h5, sin_h5, cos_h7, sin_h7]
%   A_latest : A 恢复系数（可标量或向量；向量时自动取 max(abs(.))）
%   alpha    : EMA 系数 [0,1]，建议 0.10~0.16
%   reset    : 复位信号（true 时重置 EMA 状态）
%
% 输出:
%   y_post(7x1):
%   [amp_h1_abs, amp_h3_abs, amp_h5_abs, amp_h7_abs, phase_h3, phase_h5, phase_h7]

persistent ema_state initialized
if isempty(initialized)
    ema_state = zeros(10,1,'single');
    initialized = false;
end

% -------- 参数/输入整理 --------
y = zeros(10,1,'single');
for i = 1:10
    y(i) = single(y_rel(i));
end

a = single(abs(A_latest));
if numel(a) > 1
    a = max(a(:));
end
if a < single(1e-6)
    a = single(1e-6);
end

a_ema = single(alpha);
if a_ema < single(0)
    a_ema = single(0);
elseif a_ema > single(1)
    a_ema = single(1);
end

do_reset = (reset ~= 0);

% -------- EMA --------
if ~initialized || do_reset
    ema_state = y;
    initialized = true;
else
    ema_state = a_ema * y + (single(1) - a_ema) * ema_state;
end

% -------- A 恢复（幅值）--------
amp = ema_state(1:4) * a;

% -------- 相位恢复（cos/sin -> atan2）--------
% 先单位化，避免 cos/sin 长度漂移导致相位抖动
c3 = ema_state(5); s3 = ema_state(6);
n3 = sqrt(c3*c3 + s3*s3); if n3 < single(1e-6), n3 = single(1e-6); end
c3 = c3 / n3; s3 = s3 / n3;

c5 = ema_state(7); s5 = ema_state(8);
n5 = sqrt(c5*c5 + s5*s5); if n5 < single(1e-6), n5 = single(1e-6); end
c5 = c5 / n5; s5 = s5 / n5;

c7 = ema_state(9); s7 = ema_state(10);
n7 = sqrt(c7*c7 + s7*s7); if n7 < single(1e-6), n7 = single(1e-6); end
c7 = c7 / n7; s7 = s7 / n7;

ph3 = atan2(s3, c3);
ph5 = atan2(s5, c5);
ph7 = atan2(s7, c7);

% -------- 最终输出（仅最终量）--------
y_post = zeros(7,1,'single');
y_post(1:4) = amp;
y_post(5) = ph3;
y_post(6) = ph5;
y_post(7) = ph7;

end

== matlab function PV_MEV/EV System1/PFC Control/MCP Function Half bridge1 ==
  data: i_L input; y output; i_ref input; V_in input; Ts input; L_in input; V_o input
function y = fcn(i_L, i_ref, V_in, Ts, L_in, V_o)

    L=2*pi*50*L_in;
    % --- Candidate 1: Switch ON ---
    g_on  = i_L + abs(V_in)*Ts/L;
    e_on  = abs(g_on - i_ref);

    % --- Candidate 2: Switch OFF ---
    g_off = i_L + (abs(V_in)-V_o)*Ts/L;
    e_off = abs(g_off - i_ref);

    % --- MPC Decision: pick action with lower predicted error ---
    if e_on <= e_off
        y = true;
    else
        y = false;
    end

== matlab function PV_MEV/EV System1/PFC Control/One  Cycle Model Prediction/MATLAB Function ==
  data: x input; x_norm output; A output
function [x_norm, A] = CycleNorm(x)
A = max(abs(x));
A = max(A, 1e-6);
x_norm = x / A;

== matlab function PV_MEV/EV System1/PFC Control/One  Cycle Model Prediction/MATLAB Function3 ==
  data: y_rel input; y_post output; A_latest input; alpha input; reset input
function y_post = harmonic_postprocess(y_rel, A_latest, alpha, reset)
%#codegen
% 一体化后处理：
% 1) EMA 平滑（在相对输出域）
% 2) A 恢复（幅值乘 A）
% 3) atan2 恢复相位（由 cos/sin -> phase）
%
% 输入:
%   y_rel    : 模型输出(10x1 或 1x10)
%              [amp_h1_rel, amp_h3_rel, amp_h5_rel, amp_h7_rel, ...
%               cos_h3, sin_h3, cos_h5, sin_h5, cos_h7, sin_h7]
%   A_latest : A 恢复系数（可标量或向量；向量时自动取 max(abs(.))）
%   alpha    : EMA 系数 [0,1]，建议 0.10~0.16
%   reset    : 复位信号（true 时重置 EMA 状态）
%
% 输出:
%   y_post(7x1):
%   [amp_h1_abs, amp_h3_abs, amp_h5_abs, amp_h7_abs, phase_h3, phase_h5, phase_h7]

persistent ema_state initialized
if isempty(initialized)
    ema_state = zeros(10,1,'single');
    initialized = false;
end

% -------- 参数/输入整理 --------
y = zeros(10,1,'single');
for i = 1:10
    y(i) = single(y_rel(i));
end

a = single(abs(A_latest));
if numel(a) > 1
    a = max(a(:));
end
if a < single(1e-6)
    a = single(1e-6);
end

a_ema = single(alpha);
if a_ema < single(0)
    a_ema = single(0);
elseif a_ema > single(1)
    a_ema = single(1);
end

do_reset = (reset ~= 0);

% -------- EMA --------
if ~initialized || do_reset
    ema_state = y;
    initialized = true;
else
    ema_state = a_ema * y + (single(1) - a_ema) * ema_state;
end

% -------- A 恢复（幅值）--------
amp = ema_state(1:4) * a;

% -------- 相位恢复（cos/sin -> atan2）--------
% 先单位化，避免 cos/sin 长度漂移导致相位抖动
c3 = ema_state(5); s3 = ema_state(6);
n3 = sqrt(c3*c3 + s3*s3); if n3 < single(1e-6), n3 = single(1e-6); end
c3 = c3 / n3; s3 = s3 / n3;

c5 = ema_state(7); s5 = ema_state(8);
n5 = sqrt(c5*c5 + s5*s5); if n5 < single(1e-6), n5 = single(1e-6); end
c5 = c5 / n5; s5 = s5 / n5;

c7 = ema_state(9); s7 = ema_state(10);
n7 = sqrt(c7*c7 + s7*s7); if n7 < single(1e-6), n7 = single(1e-6); end
c7 = c7 / n7; s7 = s7 / n7;

ph3 = atan2(s3, c3);
ph5 = atan2(s5, c5);
ph7 = atan2(s7, c7);

% -------- 最终输出（仅最终量）--------
y_post = zeros(7,1,'single');
y_post(1:4) = amp;
y_post(5) = ph3;
y_post(6) = ph5;
y_post(7) = ph7;

end

== matlab function PV_MEV/EV System1/PFC Control/RLS_estimation ==
  data: i_L input; amp_est output; theta_pll input; Ts input; reset input; phase_est output; i_h_est output; thdi_est output
function [amp_est, phase_est, i_h_est, thdi_est] = RLS_estimation(i_L, theta_pll, Ts, reset)
%#codegen

nParam = 9;

amp_est = zeros(4, 1);
phase_est = zeros(3, 1);
i_h_est = 0.0;
thdi_est = 0.0;

Ts_eff = max(Ts, 1e-9);

persistent w;
persistent wf;
persistent P;
persistent Ipk_filt;
persistent phase_prev;

if isempty(w) || reset ~= 0
    w = zeros(nParam, 1);
    wf = zeros(nParam, 1);
    P = zeros(nParam, nParam);

    P0 = 250.0;

    for r = 1:nParam
        for c = 1:nParam
            if r == c
                P(r, c) = P0;
            else
                P(r, c) = 0.0;
            end
        end
    end

    Ipk_filt = max(abs(i_L), 1.0);
    phase_prev = zeros(3, 1);
end

Ipk_guard = max(Ipk_filt, 1.0);

tau_est = 0.018;
lambda = exp(-Ts_eff / tau_est);

if lambda < 0.980
    lambda = 0.980;
elseif lambda > 0.99998
    lambda = 0.99998;
end

theta = atan2(sin(theta_pll), cos(theta_pll));

s1 = sin(theta);
c1 = cos(theta);

s3 = sin(3.0 * theta);
c3 = cos(3.0 * theta);

s5 = sin(5.0 * theta);
c5 = cos(5.0 * theta);

s7 = sin(7.0 * theta);
c7 = cos(7.0 * theta);

x = zeros(nParam, 1);

x(1) = 1.0;
x(2) = s1;
x(3) = c1;
x(4) = s3;
x(5) = c3;
x(6) = s5;
x(7) = c5;
x(8) = s7;
x(9) = c7;

y_hat = 0.0;

for k = 1:nParam
    y_hat = y_hat + x(k) * w(k);
end

e = i_L - y_hat;

e_lim = 0.25 * Ipk_guard;

if e_lim < 0.5
    e_lim = 0.5;
end

if e > e_lim
    e = e_lim;
elseif e < -e_lim
    e = -e_lim;
end

Px = zeros(nParam, 1);

for r = 1:nParam
    acc = 0.0;

    for c = 1:nParam
        acc = acc + P(r, c) * x(c);
    end

    Px(r) = acc;
end

xTPx = 0.0;

for k = 1:nParam
    xTPx = xTPx + x(k) * Px(k);
end

den = lambda + xTPx;

if den < 1e-9
    den = 1e-9;
end

K = zeros(nParam, 1);

for k = 1:nParam
    K(k) = Px(k) / den;
end

for k = 1:nParam
    w(k) = w(k) + K(k) * e;
end

for r = 1:nParam
    for c = 1:nParam
        P(r, c) = (P(r, c) - K(r) * Px(c)) / lambda;
    end
end

for r = 1:nParam
    for c = 1:nParam
        if c > r
            p_avg = 0.5 * (P(r, c) + P(c, r));
            P(r, c) = p_avg;
            P(c, r) = p_avg;
        end
    end
end

Pmax = 1e5;
Pmin = 1e-7;

for k = 1:nParam
    if P(k, k) > Pmax
        P(k, k) = Pmax;
    elseif P(k, k) < Pmin
        P(k, k) = Pmin;
    end
end

tau_out = 0.004;
alpha_w = 1.0 - exp(-Ts_eff / tau_out);

if alpha_w < 0.001
    alpha_w = 0.001;
elseif alpha_w > 0.10
    alpha_w = 0.10;
end

for k = 1:nParam
    wf(k) = (1.0 - alpha_w) * wf(k) + alpha_w * w(k);
end

a1 = wf(2);
b1 = wf(3);

a3 = wf(4);
b3 = wf(5);

a5 = wf(6);
b5 = wf(7);

a7 = wf(8);
b7 = wf(9);

A1 = sqrt(a1 * a1 + b1 * b1);
A3 = sqrt(a3 * a3 + b3 * b3);
A5 = sqrt(a5 * a5 + b5 * b5);
A7 = sqrt(a7 * a7 + b7 * b7);

Ipk_now = max(abs(i_L), A1);

if Ipk_now > Ipk_filt
    Ipk_filt = 0.05 * Ipk_now + 0.95 * Ipk_filt;
else
    Ipk_filt = 0.002 * Ipk_now + 0.998 * Ipk_filt;
end

Ipk = max(Ipk_filt, 1e-6);

A1_lim = 1.50 * Ipk;
A3_lim = 0.20 * Ipk;
A5_lim = 0.20 * Ipk;
A7_lim = 0.20 * Ipk;

if A1 > A1_lim
    A1 = A1_lim;
end

if A3 > A3_lim
    A3 = A3_lim;
end

if A5 > A5_lim
    A5 = A5_lim;
end

if A7 > A7_lim
    A7 = A7_lim;
end

phase_min = 0.0015 * Ipk;

if A3 > phase_min
    phi3 = atan2(b3, a3);
    phase_prev(1) = phi3;
else
    phi3 = phase_prev(1);
end

if A5 > phase_min
    phi5 = atan2(b5, a5);
    phase_prev(2) = phi5;
else
    phi5 = phase_prev(2);
end

if A7 > phase_min
    phi7 = atan2(b7, a7);
    phase_prev(3) = phi7;
else
    phi7 = phase_prev(3);
end

phi3 = atan2(sin(phi3), cos(phi3));
phi5 = atan2(sin(phi5), cos(phi5));
phi7 = atan2(sin(phi7), cos(phi7));

amp_est(1) = A1;
amp_est(2) = A3;
amp_est(3) = A5;
amp_est(4) = A7;

phase_est(1) = phi3;
phase_est(2) = phi5;
phase_est(3) = phi7;

i_h_est = a3 * s3 + b3 * c3 + a5 * s5 + b5 * c5 + a7 * s7 + b7 * c7;

if A1 > 1e-6
    thdi_est = sqrt(A3 * A3 + A5 * A5 + A7 * A7) / A1;
else
    thdi_est = 0.0;
end

end

== matlab function PV_MEV/EV System1/PFC Control/UMPC Function Full bridge1 ==
  data: i_L input; y output; i_ref input; V_in input; Ts input; L_in input; V_o input; g_on output; g_off output
function [y,g_on,g_off]= fcn(i_L, i_ref, V_in, Ts, L_in, V_o)

    L=L_in;

    if V_in >= 0
        i_ref_signed = i_ref;
    else
        i_ref_signed = -i_ref;
    end;

    % -- Positive half Cycle
    if V_in >0
        % --- Candidate 1: Switch ON ---
        g_on  = i_L + (V_in)*Ts/L;
        e_on  = abs(g_on - i_ref_signed);
        
        % --- Candidate 2: Switch OFF ---
        g_off = i_L + (V_in - V_o)*Ts/L;
        e_off = abs(g_off - i_ref_signed);

     % -- Negative half Cycle
    else
        % --- Candidate 1: Switch ON ---
        g_on  = i_L + (V_in)*Ts/L;
        e_on  = abs(g_on - i_ref_signed);

        % --- Candidate 2: Switch OFF ---
        g_off = i_L + (V_in + V_o)*Ts/L;
        e_off = abs(g_off - i_ref_signed);
    end

    % --- MPC Decision: pick action with lower predicted error ---
    if e_on <= e_off
        y = true;
    else
        y = false;
    end

== matlab function PV_MEV/EV System1/PFC Control/fft estimation 1 cycle2/FFT_estimation_1 ==
  data: u input; amp output; phase output; fs input; f0 input
function [amp, phase] = FFT_estimation_1(u, fs, f0)
%#codegen

x = double(u(:));
N = length(x);

h = zeros(4, 1);
h(1) = 1;
h(2) = 3;
h(3) = 5;
h(4) = 7;

X = fft(x);

amp = zeros(4, 1);
phase_abs_sin = zeros(4, 1);
phase = zeros(3, 1);

tol = 1e-12;

for i = 1:4
    harmonicOrder = h(i);

    bin = round(harmonicOrder * f0 * double(N) / fs);

    if bin <= 0 || bin > floor(double(N) / 2)
        amp(i) = 0;
        phase_abs_sin(i) = 0;
    else
        idx = int32(bin + 1);
        C = X(idx);

        if mod(N, 2) == 0 && bin == N / 2
            amp(i) = abs(C) / double(N);
        else
            amp(i) = 2 * abs(C) / double(N);
        end

        if amp(i) < tol
            phase_abs_sin(i) = 0;
        else
            ph_raw = angle(C);

            ph_sin = ph_raw + pi/2;

            phase_abs_sin(i) = atan2(sin(ph_sin), cos(ph_sin));
        end
    end
end

if amp(1) < tol
    phase(1) = 0;
    phase(2) = 0;
    phase(3) = 0;
else
    phase(1) = atan2( ...
        sin(phase_abs_sin(2) - 3 * phase_abs_sin(1)), ...
        cos(phase_abs_sin(2) - 3 * phase_abs_sin(1)) ...
    );

    phase(2) = atan2( ...
        sin(phase_abs_sin(3) - 5 * phase_abs_sin(1)), ...
        cos(phase_abs_sin(3) - 5 * phase_abs_sin(1)) ...
    );

    phase(3) = atan2( ...
        sin(phase_abs_sin(4) - 7 * phase_abs_sin(1)), ...
        cos(phase_abs_sin(4) - 7 * phase_abs_sin(1)) ...
    );
end

end

== matlab function PV_MEV/EV System1/PFC Control/fft estimation 10 cycle2/FFT_estimation ==
  data: u input; amp output; phase output; fs input; f0 input
function [amp, phase] = FFT_estimation(u, fs, f0)
%#codegen

x = double(u(:));
N = length(x);

h = zeros(4, 1);
h(1) = 1;
h(2) = 3;
h(3) = 5;
h(4) = 7;

X = fft(x);

amp = zeros(4, 1);
phase_abs_sin = zeros(4, 1);
phase = zeros(3, 1);

tol = 1e-12;

for i = 1:4
    harmonicOrder = h(i);

    bin = round(harmonicOrder * f0 * double(N) / fs);

    if bin <= 0 || bin > floor(double(N) / 2)
        amp(i) = 0;
        phase_abs_sin(i) = 0;
    else
        idx = int32(bin + 1);
        C = X(idx);

        if mod(N, 2) == 0 && bin == N / 2
            amp(i) = abs(C) / double(N);
        else
            amp(i) = 2 * abs(C) / double(N);
        end

        if amp(i) < tol
            phase_abs_sin(i) = 0;
        else
            ph_raw = angle(C);

            ph_sin = ph_raw + pi/2;

            phase_abs_sin(i) = atan2(sin(ph_sin), cos(ph_sin));
        end
    end
end

if amp(1) < tol
    phase(1) = 0;
    phase(2) = 0;
    phase(3) = 0;
else
    phase(1) = atan2( ...
        sin(phase_abs_sin(2) - 3 * phase_abs_sin(1)), ...
        cos(phase_abs_sin(2) - 3 * phase_abs_sin(1)) ...
    );

    phase(2) = atan2( ...
        sin(phase_abs_sin(3) - 5 * phase_abs_sin(1)), ...
        cos(phase_abs_sin(3) - 5 * phase_abs_sin(1)) ...
    );

    phase(3) = atan2( ...
        sin(phase_abs_sin(4) - 7 * phase_abs_sin(1)), ...
        cos(phase_abs_sin(4) - 7 * phase_abs_sin(1)) ...
    );
end

end
